simulink model "EE2_RetourEtat"  (R2015a)
settings: Solver=ode45  StartTime=0.0  StopTime=10.0  RelTol=1e-9
values from neighbouring files (symbols this model uses):
  K = place(EE2.ee.a, EE2.ee.b, vp_desire)    [CommandeEE2.m]    (also in CommandeEE2_RetourIntTD.m = [0 K(2)])
undefined symbols (not defined in the file or in its folder): EE1, EE2, obsver
settings Model: Creator=Lucien  LastModifiedBy=Lucien

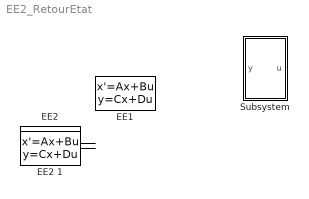
== system EE2_RetourEtat ==
  EE1 : StateSpace  A=EE1.ee.a  B=EE1.ee.b  C=EE1.ee.c  D=EE1.ee.d  X0=0
  "EE2 " : StateSpace  A=EE2.ee.a  B=EE2.ee.b  C=EE2.ee.c  D=EE2.ee.d  X0=0
  EE2 1 : StateSpace  A=EE2.ee.a  B=EE2.ee.b  C=EE2.ee.c  D=EE2.ee.d  X0=0
  Subsystem : Subsystem
  wires:
  EE2 1/1 -> ?
  "EE2 "/1 -> ?

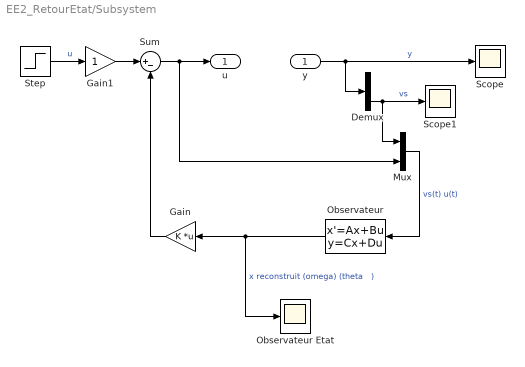
== system EE2_RetourEtat/Subsystem ==
  y : Inport
  Demux : Demux  Outputs=2
  Gain : Gain  Gain=K  Multiplication=Matrix(K*u)
  Gain1 : Gain
  Mux : Mux  Inputs=2
  "Observateur " : StateSpace  A=obsver.ee.a  B=obsver.ee.b  C=obsver.ee.c  D=obsver.ee.d  X0=0
  "Observateur Etat " : Scope
  Scope : Scope
  Scope1 : Scope
      settings: SaveName=ScopeData2
  Step : Step  Time=0  SampleTime=0
  Sum : Sum  Inputs=|+-
  u : Outport
  wires:
  Gain/1 -> Sum/2
  Sum/1 -> u/1, Mux/2
  Gain1/1 -> Sum/1
  Mux/1 -> "Observateur "/1  "vs(t) u(t)"
  "Observateur "/1 -> Gain/1, "Observateur Etat "/1  "x reconstruit (omega) (theta   )"
  Demux/2 -> Scope1/1, Mux/1  "vs"
  Step/1 -> Gain1/1  "u"
  y/1 -> Scope/1, Demux/1  "y"
